simulink model "Ghost_f34"  (Simulink 8.1)
settings: Solver=ode1  StartTime=0.0  StopTime=inf  FixedStep=Ts  MaxStep=1e-3  RelTol=1e-3
PostLoadFcn:
  | NREL_Mode=1; Ghost_init;
InitFcn:
  | NREL_Mode=1; Ghost_init;
values from neighbouring files (symbols this model uses):
  DER_REL = xlsread('DER_relay.xlsx')    [relay_settings_init.m]
  Ts = 100E-6    (= 0.0001)    [BANSHEE_init.m]    (also in Ghost_init.m)
undefined symbols (not defined in the file or in its folder): CBID, Feeder3_lib, Left, SM_UtilityService, SS_Feeder3, Stim, type, utility_service_lib, V
libraries: simulink x72, cables_lib x16, breaker_lib x14, transformer_lib x7, powerlib x7, rtlab x6, Load_lib x6, ssn_lib x4, artemis x2, PHIL_lib x2, rtio_generic_modbus x2, NREL_Diesel_Genset_lib x2
(part 1 of 3)
settings Model: ARTEMISmethode_block_infos=$$__separator__$$Ghost_f34/ARTEMIS Guide$$__separator__$$  Creator=RE25624  LastModifiedBy=hptb1  BufferReuse=off
settings SolverCC: ZeroCrossAlgorithm=Adaptive
settings DataIOCC: ExternalInput=getinputstruct(op_snapshot1)  InitialState=getstatestruct(op_snapshot1)  LimitDataPoints=off  MaxDataPoints=90060  SignalLoggingSaveFormat=Dataset  SaveOutput=off  SignalLogging=off  DSMLogging=off  SaveTime=off  OutputSaveName=result
settings OptimizationCC: BlockReduction=off  OptimizeBlockIOStorage=off  BufferReuse=off  ExpressionFolding=off  LocalBlockOutputs=off
settings DebuggingCC: MaxConsecutiveZCsMsg=warning  IgnoredZcDiagnostic=none  SolverPrmCheckMsg=none  MultiTaskRateTransMsg=warning  ParameterPrecisionLossMsg=none  FcnCallInpInsideContextMsg=EnableAllAsWarning  FrameProcessingCompatibilityMsg=error  ModelReferenceExtraNoncontSigs=warning  StrictBusMsg=Warning
settings ModelReferenceCC: UpdateModelReferenceTargets=IfOutOfDate
settings SFSimCC: SFSimEcho=off
settings GRTTargetCC: CodeReplacementLibrary=C89/C90 (ANSI)

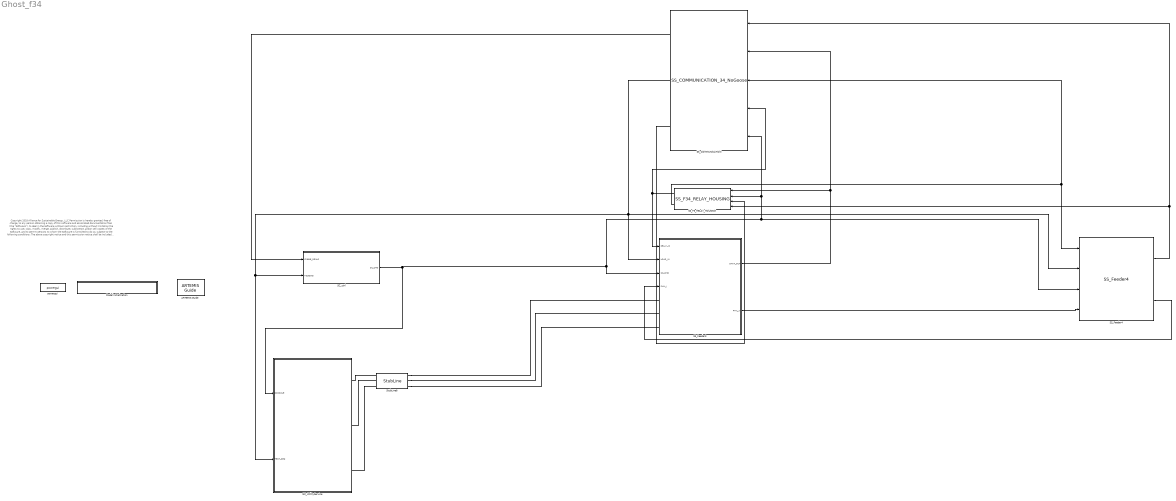
== system Ghost_f34 ==
  note: Copyright 2018 Alliance for Sustainable Energy, LLC
      |
      | Permission is hereby granted, free of charge, to any person obtaining a copy of this software
      | and associated documentation files (the "Software"), to deal in the Software without restriction,
      | including without limitation the rights to use, copy, modify, merge, publish, distribute, sublicense,
      | and/or sell copies of the Software, and to permit persons to whom the Software is furnished to do so,
      | subject to the following conditions:
      |
      | The above copyright notice and this permission notice shall be included in all copies or substantial portions of the Software.
      |
      | THE SOFTWARE IS PROVIDED "AS IS", WITHOUT WARRANTY OF ANY KIND, EXPRESS OR IMPLIED, INCLUDING
      | BUT NOT LIMITED TO THE WARRANTIES OF MERCHANTABILITY, FITNESS FOR A PARTICULAR PURPOSE AND
      | NONINFRINGEMENT. IN NO EVENT SHALL THE AUTHORS, THE COPYRIGHT HOLDERS, THE UNITED STATES,
      | THE UNITED STATES DEPARTMENT OF ENERGY, OR ANY OF THEIR EMPLOYEES BE LIABLE FOR ANY CLAIM,
      | DAMAGES OR OTHER LIABILITY, WHETHER IN AN ACTION OF CONTRACT, TORT OR OTHERWISE, ARISING FROM,
      | OUT OF OR IN CONNECTION WITH THE SOFTWARE OR THE USE OR OTHER DEALINGS IN THE SOFTWARE.
  ARTEMIS Guide : artemis/ARTEMIS/ARTEMIS Guide  Tag=FTSSmethode_opal_4hx0r99  Description=5.0_z1  lock=on  Ts=Ts  opt=art5  dyna=off  nb_perm=4  RT_fullcomp=off  ssn=on  ssn_itvc=off  ssn_ivic=off  ssn_ext=off  ssn_solver=Art5 with Backward Euler nodal interface  ssn_impulse=off  ssn_quasimpulse=off  ssn_impulse_loop=5  paraExtinctionThy=off  Thy_Impulse=on  dtc=Off  dtc_opt=normal  ao=on  simtype=off  ct_mac=off  lin_mov=off  lsp=[0.001 2]  spike_skip=Disabled  dtc_extra=1  dtc_sws=normal  dtc_pied=0.5  SPSRulesBlock=SPSRules  tre=on  ctmm=off  LF=off  dpl_type=ARTEMiS DPL  rlc_type=off  custom_type=off  para=on  ssn_ImpulseLoopBlockedStateUpdate=5  ssn_mov_iter_number=5  ssn_switch_iter_number=5  ssn_nib_type_verify=on
  Model Initialization : Subsystem  AncestorBlock=artemis/Tools /Misc/Model Initialization  mask(Model Functions){InitFcnX=NREL_Mode=1; Ghost_init;, prel=off, posl=on, inif=on, strf=off}
      mask prompts: InitFcnX "Initialisation"; prel "Preload Function"; posl "PostLoad Function"; inif "InitFcn"; strf "StartFcn"
      mask init:
      | currentBlock = gcb;
      | root = bdroot(currentBlock);
      | 
      | if ~strcmp(get_param(root,'BlockDiagramType'),'library')
      |     if prel==1
      |         set_param(root, 'PreLoadFcn', InitFcnX);
      |     else
      |         set_param(root, 'PreLoadFcn', '');
      |     end
      |     if inif==1
      |         set_param(root, 'InitFcn', InitFcnX);
      |     else
      |         set_param(root, 'InitFcn', '');
      |     end
      |     if strf==1
      |         set_param(root, 'StartFcn', InitFcnX);
      |     else
      |         set_param(root, 'StartFcn', '');
      |     end
      |     if posl==1
      |         set_param(root, 'PostLoadFcn', InitFcnX);
      |     else
      |         set_param(root, 'PostLoadFcn', '');
      |     end
      | end
      | 
      | pos = get_param(currentBlock, 'Position');
      | width = pos(3) - pos(1); height = pos(4) - pos(2);
      | txt = [ upper(root) '\n' '- InitFcn. . . . . '  get_param(root, 'InitFcn') ];
      settings: CopyFcn=set_param(gcb,'LinkStatus','inactive')
      mask Display: text(5, height*0.5, txt, 'horizontalAlignment', 'left', 'verticalAlignment', 'middle') ;
  SC_ctrl : Subsystem
  SM_UtilityService : Subsystem  AncestorBlock=utility_service_lib/SM_UtilityService
  SS_COMMUNICATION : communications_lib/SS_COMMUNICATION_34_NoGoose
  SS_F3_RELAY_HOUSING : relay_housing_lib/SS_F34_RELAY_HOUSING
  SS_Feeder3 : Subsystem  AncestorBlock=Feeder3_lib/SS_Feeder3
  SS_Feeder4 : Feeder4_lib/SS_Feeder4
  StubLine8 : artemis/ARTEMIS/StubLine  Phases=3  pu=on  L=1500 * 9.43453e-08 / 2  Lpu=0.08  R=1500 * 2.28409e-5 / 2  Rpu=0.002  S_base=50e6/3  V_base=13.8e3/sqrt(3)  F_base=60  Ts=Ts
  powergui : powerlib/powergui  Priority=2  SimulationMode=Discrete  SolverType=Tustin  SampleTime=Ts  frequency=60  SPID=off  DisableSnubberDevices=off  DisableRonSwitches=off  DisableVfSwitches=off  SwTol=0  Interpol=off  DisplayEquations=off  frequencyindice=0  Pbase=100e6  ErrMax=1e-4  Iterations=50  UnitsV=kV  UnitsW=MW  FunctionMessages=off  echomessages=off  HookPort=off  EnableUseOfTLC=off  x0status=blocks  RestoreLinks=warning  ResistiveCurrentMeasurement=off  Frange=logspace(0,3,50)  Ylog=off  Xlog=off  ShowGrid=off  save=off  variable=ZData  structure=0  ZoomFFT=on  StartTime=0.0  cycles=2  DisplayStyle=off  fundamental=60  FreqAxis=off  MaxFrequency=1000  frequencyindicesteady=1  RmsSteady=1  display=off  Ts=0  methode=off
  wires:
  SS_Feeder3/1(DATA_OUT) -> SS_COMMUNICATION/2, SS_F3_RELAY_HOUSING/1
  SS_F3_RELAY_HOUSING/1 -> SS_COMMUNICATION/4, SS_Feeder3/1(RELAY_IN)
  SS_COMMUNICATION/1 -> SC_ctrl/1(CMBNE_SGNLS)
  SC_ctrl/1(SC_CMD) -> SS_Feeder3/3(SC_CMD), SS_Feeder4/3, SS_COMMUNICATION/5, SS_F3_RELAY_HOUSING/2, SM_UtilityService/1(CONSOLE)
  SS_F3_RELAY_HOUSING/2 -> SS_COMMUNICATION/3, SS_Feeder4/1
  SS_Feeder4/1 -> SS_COMMUNICATION/1, SS_F3_RELAY_HOUSING/4
  SS_Feeder3/2(PHIL_V) -> SS_Feeder4/4
  SS_Feeder4/2 -> SS_Feeder3/4(PHIL_I)
  SS_COMMUNICATION/3 -> SS_F3_RELAY_HOUSING/3
  SS_COMMUNICATION/2 -> SS_Feeder3/2(LOAD_IN), SM_UtilityService/2(TEST_SEQ), SC_ctrl/2(TestData), SS_Feeder4/2
  connections:
  StubLine8/LConn1 -- SM_UtilityService/RConn1
  StubLine8/LConn2 -- SM_UtilityService/RConn2
  StubLine8/LConn3 -- SM_UtilityService/RConn3
  StubLine8/RConn3 -- SS_Feeder3/LConn3
  StubLine8/RConn2 -- SS_Feeder3/LConn2
  StubLine8/RConn1 -- SS_Feeder3/LConn1

== system Ghost_f34/Model Initialization ==

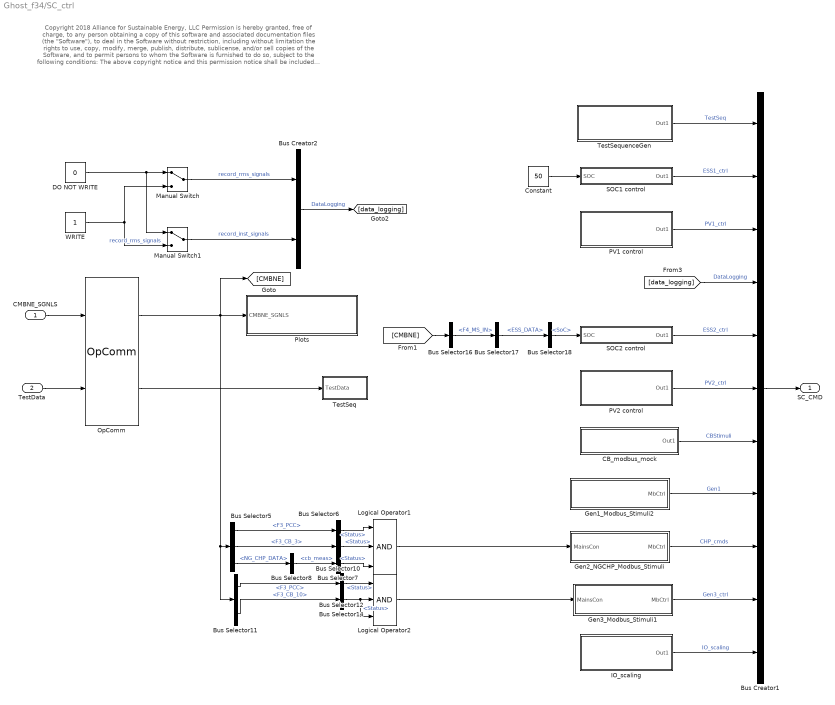
== system Ghost_f34/SC_ctrl ==
  note: Copyright 2018 Alliance for Sustainable Energy, LLC
      |
      | Permission is hereby granted, free of charge, to any person obtaining a copy of this software
      | and associated documentation files (the "Software"), to deal in the Software without restriction,
      | including without limitation the rights to use, copy, modify, merge, publish, distribute, sublicense,
      | and/or sell copies of the Software, and to permit persons to whom the Software is furnished to do so,
      | subject to the following conditions:
      |
      | The above copyright notice and this permission notice shall be included in all copies or substantial portions of the Software.
      |
      | THE SOFTWARE IS PROVIDED "AS IS", WITHOUT WARRANTY OF ANY KIND, EXPRESS OR IMPLIED, INCLUDING
      | BUT NOT LIMITED TO THE WARRANTIES OF MERCHANTABILITY, FITNESS FOR A PARTICULAR PURPOSE AND
      | NONINFRINGEMENT. IN NO EVENT SHALL THE AUTHORS, THE COPYRIGHT HOLDERS, THE UNITED STATES,
      | THE UNITED STATES DEPARTMENT OF ENERGY, OR ANY OF THEIR EMPLOYEES BE LIABLE FOR ANY CLAIM,
      | DAMAGES OR OTHER LIABILITY, WHETHER IN AN ACTION OF CONTRACT, TORT OR OTHERWISE, ARISING FROM,
      | OUT OF OR IN CONNECTION WITH THE SOFTWARE OR THE USE OR OTHER DEALINGS IN THE SOFTWARE.
  CMBNE_SGNLS : Inport
  TestData : Inport  Port=2
  Bus Creator1 : BusCreator  Inputs=11
  Bus Creator2 : BusCreator  Inputs=2
  Bus Selector{6..7,10,12,14} (5 alike) : BusSelector  OutputSignals=Status
  Bus Selector11 : BusSelector  OutputSignals=F3_MS_IN.CB_DATA.F3_PCC,F3_MS_IN.CB_DATA.F3_CB_10
  Bus Selector16 : BusSelector  OutputSignals=F4_MS_IN
  Bus Selector17 : BusSelector  OutputSignals=ESS_DATA
  Bus Selector18 : BusSelector  OutputSignals=Battery.SoC
  Bus Selector5 : BusSelector  OutputSignals=F3_MS_IN.CB_DATA.F3_PCC,F3_MS_IN.CB_DATA.F3_CB_3,F3_MS_IN.NG_CHP_DATA
  Bus Selector8 : BusSelector  OutputSignals=cb.cb_meas
  CB_modbus_mock : Subsystem
  Constant : Constant  Value=50
  DO NOT WRITE : Constant  Value=0
  Gen1_Modbus_Stimuli2 : Subsystem
  Gen2_NGCHP_Modbus_Stimuli : Subsystem
  Gen3_Modbus_Stimuli1 : Subsystem
  IO_scaling : Subsystem
  Logical Operator1 : Logic  Inputs=3  AllPortsSameDT=off  OutDataTypeStr=boolean
  Logical Operator2 : Logic  Inputs=3  AllPortsSameDT=off  OutDataTypeStr=boolean
  Manual Switch : ManualSwitch
  Manual Switch1 : ManualSwitch
  OpComm : rtlab/OpComm  nbport=2  groupe_acq=1  subsys_rate=0  st=0  Synchronization=on  Interpolation=on  Threshold=1.0  Missed_Data=off  Sim_Time=off  Samples=off  dynSigOut=off  from_console=0  warning_done=off  writeOpCommFile=off  Offset=off
  PV1 control : Subsystem
  PV2 control : Subsystem
  Plots : Subsystem
  SOC1 control : Subsystem
  SOC2 control : Subsystem
  TestSeq : Subsystem
  TestSequenceGen : Subsystem
  WRITE : Constant
  SC_CMD : Outport
  wires:
  CMBNE_SGNLS/1 -> OpComm/1
  Bus Creator1/1 -> SC_CMD/1
  Manual Switch/1 -> Bus Creator2/1  "record_rms_signals"
  Manual Switch1/1 -> Bus Creator2/2  "record_inst_signals"
  Bus Creator2/1 -> [data_logging]  "DataLogging"
  TestData/1 -> OpComm/2
  WRITE/1 -> Manual Switch1/2, Manual Switch/2  "record_rms_signals"
  DO NOT WRITE/1 -> Manual Switch1/1, Manual Switch/1
  [data_logging] -> Bus Creator1/4  "DataLogging"
  CB_modbus_mock/1(Out1) -> Bus Creator1/7  "CBStimuli"
  Gen1_Modbus_Stimuli2/1(MbCtrl) -> Bus Creator1/8  "Gen1"
  SOC2 control/1(Out1) -> Bus Creator1/5  "ESS2_ctrl"
  PV2 control/1(Out1) -> Bus Creator1/6  "PV2_ctrl"
  OpComm/1 -> [CMBNE], Bus Selector11/1, Bus Selector5/1, Plots/1(CMBNE_SGNLS)
  Gen2_NGCHP_Modbus_Stimuli/1(MbCtrl) -> Bus Creator1/9  "CHP_cmds"
  Bus Selector5/1 -> Bus Selector6/1  "<F3_PCC>"
  Bus Selector5/3 -> Bus Selector8/1  "<NG_CHP_DATA>"
  Bus Selector6/1 -> Logical Operator1/1  "<Status>"
  Bus Selector7/1 -> Logical Operator1/3  "<Status>"
  Bus Selector8/1 -> Bus Selector7/1  "<cb_meas>"
  Logical Operator1/1 -> Gen2_NGCHP_Modbus_Stimuli/1(MainsCon)
  Bus Selector10/1 -> Logical Operator1/2  "<Status>"
  Bus Selector5/2 -> Bus Selector10/1  "<F3_CB_3>"
  Gen3_Modbus_Stimuli1/1(MbCtrl) -> Bus Creator1/10  "Gen3_ctrl"
  Logical Operator2/1 -> Gen3_Modbus_Stimuli1/1(MainsCon)
  Bus Selector11/1 -> Bus Selector12/1  "<F3_PCC>"
  Bus Selector12/1 -> Logical Operator2/1  "<Status>"
  Bus Selector11/2 -> Bus Selector14/1  "<F3_CB_10>"
  Bus Selector14/1 -> Logical Operator2/3, Logical Operator2/2  "<Status>"
  OpComm/2 -> TestSeq/1(TestData)
  IO_scaling/1(Out1) -> Bus Creator1/11  "IO_scaling"
  TestSequenceGen/1(Out1) -> Bus Creator1/1  "TestSeq"
  SOC1 control/1(Out1) -> Bus Creator1/2  "ESS1_ctrl"
  PV1 control/1(Out1) -> Bus Creator1/3  "PV1_ctrl"
  Constant/1 -> SOC1 control/1(SOC)
  [CMBNE] -> Bus Selector16/1
  Bus Selector16/1 -> Bus Selector17/1  "<F4_MS_IN>"
  Bus Selector17/1 -> Bus Selector18/1  "<ESS_DATA>"
  Bus Selector18/1 -> SOC2 control/1(SOC)  "<SoC>"

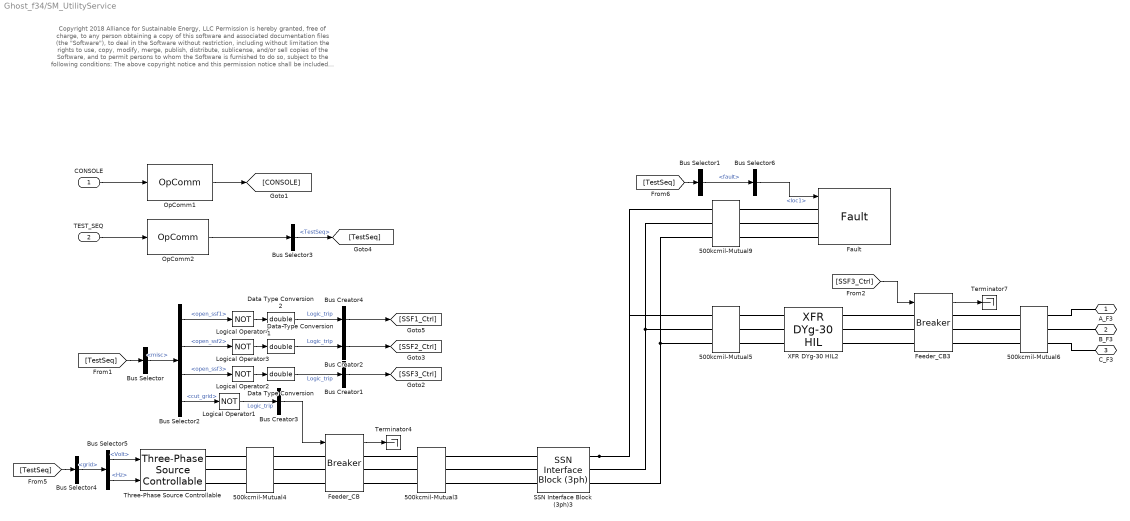
== system Ghost_f34/SM_UtilityService ==
  note: Copyright 2018 Alliance for Sustainable Energy, LLC
      |
      | Permission is hereby granted, free of charge, to any person obtaining a copy of this software
      | and associated documentation files (the "Software"), to deal in the Software without restriction,
      | including without limitation the rights to use, copy, modify, merge, publish, distribute, sublicense,
      | and/or sell copies of the Software, and to permit persons to whom the Software is furnished to do so,
      | subject to the following conditions:
      |
      | The above copyright notice and this permission notice shall be included in all copies or substantial portions of the Software.
      |
      | THE SOFTWARE IS PROVIDED "AS IS", WITHOUT WARRANTY OF ANY KIND, EXPRESS OR IMPLIED, INCLUDING
      | BUT NOT LIMITED TO THE WARRANTIES OF MERCHANTABILITY, FITNESS FOR A PARTICULAR PURPOSE AND
      | NONINFRINGEMENT. IN NO EVENT SHALL THE AUTHORS, THE COPYRIGHT HOLDERS, THE UNITED STATES,
      | THE UNITED STATES DEPARTMENT OF ENERGY, OR ANY OF THEIR EMPLOYEES BE LIABLE FOR ANY CLAIM,
      | DAMAGES OR OTHER LIABILITY, WHETHER IN AN ACTION OF CONTRACT, TORT OR OTHERWISE, ARISING FROM,
      | OUT OF OR IN CONNECTION WITH THE SOFTWARE OR THE USE OR OTHER DEALINGS IN THE SOFTWARE.
  CONSOLE : Inport
  TEST_SEQ : Inport  Port=2
  500kcmil-Mutual3 : cables_lib/500kcmil-Mutual  length=50  par_sets=1  ratio=3
  500kcmil-Mutual4 : cables_lib/500kcmil-Mutual  length=50  par_sets=1  ratio=3
  500kcmil-Mutual5 : cables_lib/500kcmil-Mutual  length=200  par_sets=1  ratio=3
  500kcmil-Mutual6 : cables_lib/500kcmil-Mutual  length=50  par_sets=1  ratio=3
  500kcmil-Mutual9 : cables_lib/500kcmil-Mutual  length=200  par_sets=1  ratio=3
  Bus Creator{1..4} (4 alike) : BusCreator  Inputs=1
  Bus Selector : BusSelector  OutputSignals=misc
  Bus Selector1 : BusSelector  OutputSignals=fault
  Bus Selector2 : BusSelector  OutputSignals=open_ssf1,open_ssf2,open_ssf3,cut_grid
  Bus Selector3 : BusSelector  OutputSignals=TestSeq
  Bus Selector4 : BusSelector  OutputSignals=grid
  Bus Selector5 : BusSelector  OutputSignals=Volt,Hz
  Bus Selector6 : BusSelector  OutputSignals=loc1
  Data Type Conversion : DataTypeConversion  OutDataTypeStr=double
  Data Type Conversion1 : DataTypeConversion  OutDataTypeStr=double
  Data Type Conversion2 : DataTypeConversion  OutDataTypeStr=double
  Fault : fault_lib/Fault  FaultResistance=0.1  GroundResistance=1.73  SnubberResistance=1E6
  Feeder_CB : breaker_lib/Breaker  Ts=Ts  mech_delay=cb_mech_delay
  Feeder_CB3 : breaker_lib/Breaker  Ts=Ts  mech_delay=cb_mech_delay
  Logical Operator{1..4} (4 alike) : Logic  Operator=NOT  AllPortsSameDT=off  OutDataTypeStr=boolean
  OpComm1 : rtlab/OpComm  nbport=1  groupe_acq=1  subsys_rate=0  st=0  Synchronization=on  Interpolation=on  Threshold=1.0  Missed_Data=off  Sim_Time=off  Samples=off  dynSigOut=off  from_console=1  warning_done=off  writeOpCommFile=off  Offset=off
  OpComm2 : rtlab/OpComm  nbport=1  groupe_acq=1  subsys_rate=0  st=0  Synchronization=on  Interpolation=on  Threshold=1.0  Missed_Data=off  Sim_Time=off  Samples=off  dynSigOut=off  from_console=0  warning_done=off  writeOpCommFile=off  Offset=off
  SSN Interface Block (3ph)3 : ssn_lib/SSN Interface Block (3ph)  nb_phase=3  nb_port=2  p1_type=V-type(Left)  p2_type=V-type (Right)  p3_type=V-type(Left)  p4_type=V-type(Left)  p5_type=V-type(Left)  p6_type=V-type(Left)  p7_type=V-type(Left)  p8_type=V-type(Left)  p9_type=V-type(Left)  p10_type=V-type(Left)  p11_type=V-type(Left)  p12_type=V-type(Left)  p13_type=V-type(Left)  p14_type=V-type(Left)  p15_type=V-type(Left)  p16_type=V-type(Left)  I_port_shunt_resistance=1e9
  Terminator4 : Terminator
  Terminator7 : Terminator
  Three-Phase Source Controllable : controllable_grid_lib/Three-Phase Source Controllable  Ts=Ts  Rg=0.8  Lg=16.58e-3  mask{Ts=Ts}
  XFR DYg-30 HIL2 : transformer_lib/XFR DYg-30 HIL  Rating=50000  Vp=115000  Vs=13800  Z=6  XR=30
  A_F3 : PMIOPort  Port=1  Side=Right
  B_F3 : PMIOPort  Port=2  Side=Right
  C_F3 : PMIOPort  Port=3  Side=Right
  wires:
  CONSOLE/1 -> OpComm1/1
  OpComm1/1 -> [CONSOLE]
  Feeder_CB/1 -> Terminator4/1
  Feeder_CB3/1 -> Terminator7/1
  TEST_SEQ/1 -> OpComm2/1
  [TestSeq] -> Bus Selector/1
  Logical Operator1/1 -> Bus Creator3/1  "Logic_trip"
  Bus Creator3/1 -> Feeder_CB/1
  Bus Selector/1 -> Bus Selector2/1  "<misc>"
  Bus Selector2/4 -> Logical Operator1/1  "<cut_grid>"
  Bus Selector2/3 -> Logical Operator2/1  "<open_ssf3>"
  Logical Operator2/1 -> Data Type Conversion/1
  Bus Creator1/1 -> [SSF3_Ctrl]
  Data Type Conversion/1 -> Bus Creator1/1  "Logic_trip"
  Bus Selector3/1 -> [TestSeq]  "<TestSeq>"
  OpComm2/1 -> Bus Selector3/1
  Bus Selector2/2 -> Logical Operator3/1  "<open_ssf2>"
  Logical Operator3/1 -> Data Type Conversion1/1
  Bus Creator2/1 -> [SSF2_Ctrl]
  Data Type Conversion1/1 -> Bus Creator2/1  "Logic_trip"
  Bus Selector2/1 -> Logical Operator4/1  "<open_ssf1>"
  Logical Operator4/1 -> Data Type Conversion2/1
  Bus Creator4/1 -> [SSF1_Ctrl]
  Data Type Conversion2/1 -> Bus Creator4/1  "Logic_trip"
  [SSF3_Ctrl] -> Feeder_CB3/1
  [TestSeq] -> Bus Selector4/1
  Bus Selector4/1 -> Bus Selector5/1  "<grid>"
  Bus Selector5/2 -> Three-Phase Source Controllable/2  "<Hz>"
  Bus Selector5/1 -> Three-Phase Source Controllable/1  "<Volt>"
  [TestSeq] -> Bus Selector1/1
  Bus Selector1/1 -> Bus Selector6/1  "<fault>"
  Bus Selector6/1 -> Fault/1  "<loc1>"
  connections:
  500kcmil-Mutual3/LConn3 -- Feeder_CB/RConn3
  500kcmil-Mutual3/LConn1 -- Feeder_CB/RConn1
  500kcmil-Mutual3/LConn2 -- Feeder_CB/RConn2
  SSN Interface Block (3ph)3/LConn2 -- 500kcmil-Mutual3/RConn2
  SSN Interface Block (3ph)3/LConn1 -- 500kcmil-Mutual3/RConn1
  SSN Interface Block (3ph)3/LConn3 -- 500kcmil-Mutual3/RConn3
  500kcmil-Mutual4/RConn3 -- Feeder_CB/LConn3
  500kcmil-Mutual4/RConn2 -- Feeder_CB/LConn2
  500kcmil-Mutual4/RConn1 -- Feeder_CB/LConn1
  Three-Phase Source Controllable/RConn3 -- 500kcmil-Mutual4/LConn3
  Three-Phase Source Controllable/RConn1 -- 500kcmil-Mutual4/LConn1
  Three-Phase Source Controllable/RConn2 -- 500kcmil-Mutual4/LConn2
  500kcmil-Mutual5/RConn2 -- XFR DYg-30 HIL2/LConn2
  500kcmil-Mutual5/RConn1 -- XFR DYg-30 HIL2/LConn1
  500kcmil-Mutual5/RConn3 -- XFR DYg-30 HIL2/LConn3
  SSN Interface Block (3ph)3/RConn1 -- 500kcmil-Mutual5/LConn1 -- 500kcmil-Mutual9/LConn1
  500kcmil-Mutual5/LConn2 -- SSN Interface Block (3ph)3/RConn2 -- 500kcmil-Mutual9/LConn2
  500kcmil-Mutual5/LConn3 -- SSN Interface Block (3ph)3/RConn3 -- 500kcmil-Mutual9/LConn3
  XFR DYg-30 HIL2/RConn1 -- Feeder_CB3/LConn1
  XFR DYg-30 HIL2/RConn2 -- Feeder_CB3/LConn2
  XFR DYg-30 HIL2/RConn3 -- Feeder_CB3/LConn3
  500kcmil-Mutual6/LConn2 -- Feeder_CB3/RConn2
  500kcmil-Mutual6/LConn3 -- Feeder_CB3/RConn3
  500kcmil-Mutual6/LConn1 -- Feeder_CB3/RConn1
  B_F3/RConn1 -- 500kcmil-Mutual6/RConn2
  A_F3/RConn1 -- 500kcmil-Mutual6/RConn1
  C_F3/RConn1 -- 500kcmil-Mutual6/RConn3
  500kcmil-Mutual9/RConn2 -- Fault/LConn2
  500kcmil-Mutual9/RConn3 -- Fault/LConn3
  500kcmil-Mutual9/RConn1 -- Fault/LConn1

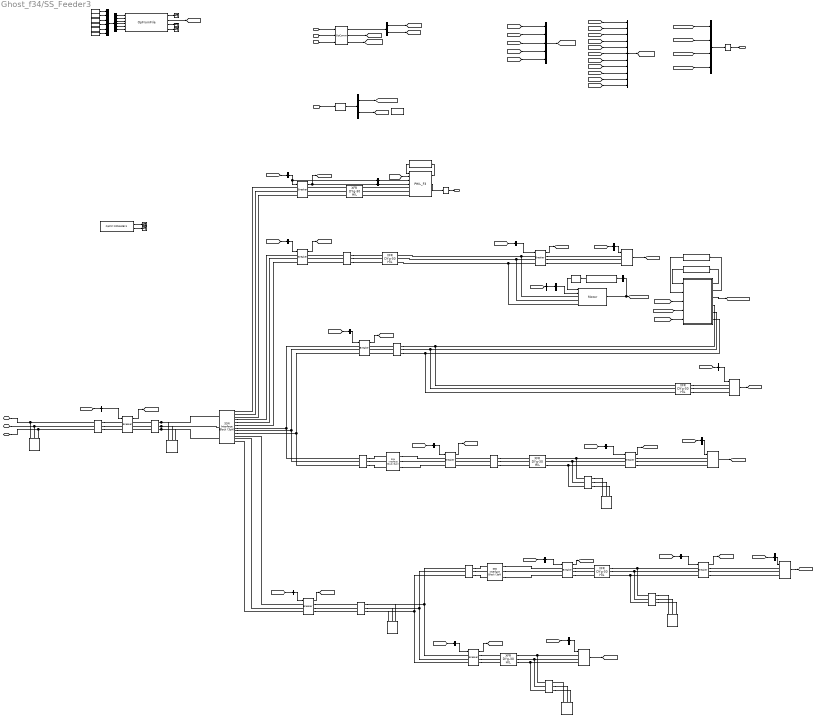
== system Ghost_f34/SS_Feeder3 ==
  note: Signal for this Cb will come from a SEL relay
  note: connect to F2
  note: connect to F2
  note: PHIL interface
  note: Copyright 2018 Alliance for Sustainable Energy, LLC
      |
      | Permission is hereby granted, free of charge, to any person obtaining a copy of this software
      | and associated documentation files (the "Software"), to deal in the Software without restriction,
      | including without limitation the rights to use, copy, modify, merge, publish, distribute, sublicense,
      | and/or sell copies of the Software, and to permit persons to whom the Software is furnished to do so,
      | subject to the following conditions:
      |
      | The above copyright notice and this permission notice shall be included in all copies or substantial portions of the Software.
      |
      | THE SOFTWARE IS PROVIDED "AS IS", WITHOUT WARRANTY OF ANY KIND, EXPRESS OR IMPLIED, INCLUDING
      | BUT NOT LIMITED TO THE WARRANTIES OF MERCHANTABILITY, FITNESS FOR A PARTICULAR PURPOSE AND
      | NONINFRINGEMENT. IN NO EVENT SHALL THE AUTHORS, THE COPYRIGHT HOLDERS, THE UNITED STATES,
      | THE UNITED STATES DEPARTMENT OF ENERGY, OR ANY OF THEIR EMPLOYEES BE LIABLE FOR ANY CLAIM,
      | DAMAGES OR OTHER LIABILITY, WHETHER IN AN ACTION OF CONTRACT, TORT OR OTHERWISE, ARISING FROM,
      | OUT OF OR IN CONNECTION WITH THE SOFTWARE OR THE USE OR OTHER DEALINGS IN THE SOFTWARE.
  RELAY_IN : Inport
  LOAD_IN : Inport  Port=2
  SC_CMD : Inport  Port=3
  PHIL_I : Inport  Port=4
  1000 kVA : transformer_lib/XFR DYg-30 HIL  Rating=1000  Vp=13800  Vs=480  Z=5.56  XR=5.49
  1000 kVA1 : transformer_lib/XFR DYg-30 HIL  Rating=1000  Vp=13800  Vs=480  Z=5.56  XR=5.49
  200 HP chiller compressor : Load_lib/200 HP chiller compressor
  2000 kVA : transformer_lib/XFR DYg-30 HIL  Rating=2000  Vp=13800  Vs=480  Z=5.75  XR=5.7
  2000 kVA1 : transformer_lib/XFR DYg-30 HIL  Rating=2000  Vp=13800  Vs=480  Z=5.75  XR=5.7
  2500 kVA : transformer_lib/XFR DYg-30 HIL  Rating=2500  Vp=13800  Vs=480  Z=5.75  XR=6.6
  2500 kVA1 : transformer_lib/XFR DYg-30 HIL  Rating=5000  Vp=13800  Vs=4160  Z=5.75  XR=6.6
  448 kvar inductor at 13.8kV  to cancel kvar produced by the stublines1 : powerlib/Elements/Three-Phase Parallel RLC Load  LConnTagsString=A|B|C  Configuration=Y (grounded)  NominalVoltage=13800  NominalFrequency=60  ActivePower=10e3  InductivePower=448e3  CapacitivePower=0  Measurements=None  LoadType=constant Z
  500kcmil-Mutual1 : cables_lib/500kcmil-Mutual  length=10  par_sets=1  ratio=3
  500kcmil-Mutual2 : cables_lib/500kcmil-Mutual  length=10  par_sets=1  ratio=3
  500kcmil-Mutual3 : cables_lib/500kcmil-Mutual  length=100  par_sets=1  ratio=3
  500kcmil-Mutual4 : cables_lib/500kcmil-Mutual  length=10  par_sets=1  ratio=3
  500kcmil-Mutual5 : cables_lib/500kcmil-Mutual  length=1000  par_sets=1  ratio=3
  6 kvar inductor at 480V  to cancel kvar produced by the stublines1 : powerlib/Elements/Three-Phase Parallel RLC Load  LConnTagsString=A|B|C  Configuration=Y (grounded)  NominalVoltage=480  NominalFrequency=60  ActivePower=1e3  InductivePower=6e3  CapacitivePower=0  Measurements=None  LoadType=constant Z
  6 kvar inductor at 480V  to cancel kvar produced by the stublines2 : powerlib/Elements/Three-Phase Parallel RLC Load  LConnTagsString=A|B|C  Configuration=Y (grounded)  NominalVoltage=480  NominalFrequency=60  ActivePower=1e3  InductivePower=6e3  CapacitivePower=0  Measurements=None  LoadType=constant Z
  6 kvar inductor at 480V  to cancel kvar produced by the stublines3 : powerlib/Elements/Three-Phase Parallel RLC Load  LConnTagsString=A|B|C  Configuration=Y (grounded)  NominalVoltage=480  NominalFrequency=60  ActivePower=0  InductivePower=6e3  CapacitivePower=0  Measurements=None  LoadType=constant Z
  AIN_AOUT_OP5142EX1 : PHIL_lib/AIN_AOUT_OP5142EX1
  Bus Creator2 : BusCreator
  Bus Creator3 : BusCreator  Inputs=5
  Bus Creator5 : BusCreator  Inputs=11
  Bus Selector : BusSelector  OutputSignals=motor
  Bus Selector1 : BusSelector  OutputSignals=F3_CB_4
  Bus Selector10 : BusSelector  OutputSignals=F3_CB_5
  Bus Selector11 : BusSelector  OutputSignals=P6
  Bus Selector12 : BusSelector  OutputSignals=F3_CB_9
  Bus Selector13 : BusSelector  OutputSignals=F3_CB_3
  Bus Selector14 : BusSelector  OutputSignals=F3_CB_8
  Bus Selector15 : BusSelector  OutputSignals=CHP_cmds,IO_scaling
  Bus Selector16 : BusSelector  OutputSignals=Status
  Bus Selector17 : BusSelector  OutputSignals=RPM
  Bus Selector18 : BusSelector  OutputSignals=LoadProfile,TestSeq
  Bus Selector19 : BusSelector  OutputSignals=Logic_trip
  Bus Selector2 : BusSelector  OutputSignals=C6
  Bus Selector20 : BusSelector  OutputSignals=ena2
  Bus Selector21 : BusSelector  OutputSignals=F3_PCC
  Bus Selector22 : BusSelector  OutputSignals=F3_CB_10
  Bus Selector3 : BusSelector  OutputSignals=P4
  Bus Selector4 : BusSelector  OutputSignals=I6
  Bus Selector5 : BusSelector  OutputSignals=C5
  Bus Selector6 : BusSelector  OutputSignals=F3_CB_2
  Bus Selector7 : BusSelector  OutputSignals=F3_CB_7
  Bus Selector8 : BusSelector  OutputSignals=F3_CB_6
  Bus Selector9 : BusSelector  OutputSignals=F3_CB_1
  C1 : cables_lib/500kcmil-Mutual  length=10  par_sets=1  ratio=3
  C2 : cables_lib/500kcmil-Mutual  length=10  par_sets=1  ratio=3
  C301 : cables_lib/500kcmil-Mutual  length=2500  par_sets=1  ratio=3
  C302 : cables_lib/4//0AWG-Mutual  length=2000  par_sets=1  ratio=3
  C303 : cables_lib/500kcmil-Mutual  length=2000  par_sets=1  ratio=3
  C304 : cables_lib/4//0AWG-Mutual  length=1500  par_sets=2  ratio=3
  CHP_Modbus : rtio_generic_modbus/Modbus device  conf_name=CHP_modbus.opal  conf_name_mask=CHP_modbus.xls  sample_time=Ts
  Critical_5 : Load_lib/Dynamic_Load  V=480  kVA=1000  PF=0.9  Ts=Ts
  Critical_6 : Load_lib/Dynamic_Load  V=480  kVA=800  PF=0.9  Ts=Ts
  Demux2 : Demux  Outputs=6
  F3_CB_{1..6,8..11} (10 alike) : breaker_lib/Breaker  Ts=Ts  mech_delay=cb_mech_delay
  F3_PCC : breaker_lib/Breaker  Ts=Ts  mech_delay=cb_mech_delay
  First-Order Filter : powerlib_meascontrol/Filters/First-Order Filter  FilterType=Lowpass  Tc=10e-3  Ts=Ts  Initialize=on  Vac_Init=[0, 0, 60]  Vdc_Init=0  PlotResponse=off  FreqRange="[0,  200,  1]"
  GEN2_Modbus : rtio_generic_modbus/Modbus device  conf_name=GEN2_modbus.opal  conf_name_mask=GEN2_modbus.xls  sample_time=Ts
  Goto Tag Visibility : GotoTagVisibility  GotoTag=phil_ctrl
  "Interpolation " : Constant
  Interruptible_6 : Load_lib/Dynamic_Load  V=480  kVA=600  PF=0.9  Ts=Ts
  Losses1 : powerlib/Elements/Three-Phase Parallel RLC Load  LConnTagsString=A|B|C  Configuration=Y (grounded)  NominalVoltage=13800  NominalFrequency=60  ActivePower=1e3  InductivePower=0  CapacitivePower=0  Measurements=None  LoadType=constant Z
  Losses4 : powerlib/Elements/Three-Phase Parallel RLC Load  LConnTagsString=A|B|C  Configuration=Y (grounded)  NominalVoltage=13800  NominalFrequency=60  ActivePower=1e3  InductivePower=0  CapacitivePower=0  Measurements=None  LoadType=constant Z
  Memory : Memory
  Memory1 : Memory
  Motor : Motor_InductionMachine_lib/Motor
  Mux : Mux  Inputs=6
  NGCHP_Generator : Subsystem
  OpComm1 : rtlab/OpComm  nbport=3  groupe_acq=1  subsys_rate=0  st=0  Synchronization=on  Interpolation=on  Threshold=1.0  Missed_Data=off  Sim_Time=off  Samples=off  dynSigOut=off  from_console=0  warning_done=off  writeOpCommFile=off  Offset=off
  OpComm2 : rtlab/OpComm  nbport=1  groupe_acq=1  subsys_rate=0  st=0  Synchronization=on  Interpolation=on  Threshold=1.0  Missed_Data=off  Sim_Time=off  Samples=off  dynSigOut=off  from_console=1  warning_done=off  writeOpCommFile=off  Offset=off
  OpCtrl OP5142EX1 : rtio_opalrt_op5142ex1/OpCtrl OP5142EX1  CtrlName='OP5142EX1 Ctrl'  boardid=0  BitstreamFilename=OP5142_1-EX-0000-2_1-96IO-04-01.bin  numconfig=-1  mode=Master  externalClock=off  decimRtsi=0  calibIO=off  SampleTime=0  loadinport=-1
  OpFromFile : rtlab/DataLogging/OpFromFile  filename_mode=Static (same filename all the time)  reload_mode=Next time model is paused (Real-Time)  init_file_id=0  filename=HeatLoad.mat  rtpath='./'  nrtpath='.\'  sample_time=Ts
  PHIL_F3 : PHIL_lib/PHIL_F3
  Priority_4 : Load_lib/Dynamic_Load  V=480  kVA=600  PF=0.9  Ts=Ts
  Priority_6 : Load_lib/Dynamic_Load  V=480  kVA=1000  PF=0.9  Ts=Ts
  "Repetative " : Constant
  SSN Interface Block (3ph)1 : ssn_lib/SSN Interface Block (3ph)  nb_phase=3  nb_port=2  p1_type=V-type(Left)  p2_type=V-type (Right)  p3_type=V-type(Left)  p4_type=V-type(Left)  p5_type=V-type(Left)  p6_type=V-type(Left)  p7_type=V-type(Left)  p8_type=V-type(Left)  p9_type=V-type(Left)  p10_type=V-type(Left)  p11_type=V-type(Left)  p12_type=V-type(Left)  p13_type=V-type(Left)  p14_type=V-type(Left)  p15_type=V-type(Left)  p16_type=V-type(Left)  I_port_shunt_resistance=1e9
  SSN Interface Block (3ph)2 : ssn_lib/SSN Interface Block (3ph)  nb_phase=3  nb_port=2  p1_type=V-type(Left)  p2_type=V-type (Right)  p3_type=V-type(Left)  p4_type=V-type(Left)  p5_type=V-type(Left)  p6_type=V-type(Left)  p7_type=V-type(Left)  p8_type=V-type(Left)  p9_type=V-type(Left)  p10_type=V-type(Left)  p11_type=V-type(Left)  p12_type=V-type(Left)  p13_type=V-type(Left)  p14_type=V-type(Left)  p15_type=V-type(Left)  p16_type=V-type(Left)  I_port_shunt_resistance=1e9
  SSN Interface Block (3ph)5 : ssn_lib/SSN Interface Block (3ph)  nb_phase=3  nb_port=5  p1_type=V-type(Left)  p2_type=V-type (Right)  p3_type=V-type (Right)  p4_type=V-type (Right)  p5_type=V-type (Right)  p6_type=V-type(Left)  p7_type=V-type(Left)  p8_type=V-type(Left)  p9_type=V-type(Left)  p10_type=V-type(Left)  p11_type=V-type(Left)  p12_type=V-type(Left)  p13_type=V-type(Left)  p14_type=V-type(Left)  p15_type=V-type(Left)  p16_type=V-type(Left)  I_port_shunt_resistance=1e9
  "Start_Index " : Constant
  "State " : Constant
  "Stop_Index " : Constant  Value=1800-1
  Terminator{,1..4} (5 alike) : Terminator
  "Time_Scale_Factor " : Constant
  PCC_A : PMIOPort  Port=1  Side=Left
  PCC_B : PMIOPort  Port=2  Side=Left
  PCC_C : PMIOPort  Port=3  Side=Left
  DATA_OUT : Outport
  PHIL_V : Outport  Port=2
  tag scope: phil_ctrl=scoped
  wires:
  Bus Selector1/1 -> F3_CB_4/1  "<F3_CB_4>"
  LOAD_IN/1 -> OpComm1/1
  OpComm1/1 -> Bus Selector18/1
  [LOAD_IN] -> Bus Selector2/1
  [LOAD_IN] -> Bus Selector3/1
  [LOAD_IN] -> Bus Selector4/1
  [LOAD_IN] -> Bus Selector5/1
  Bus Selector2/1 -> Critical_6/1  "<C6>"
  Bus Selector3/1 -> Priority_4/1  "<P4>"
  Bus Selector4/1 -> Interruptible_6/1  "<I6>"
  Bus Selector5/1 -> Critical_5/1  "<C5>"
  Critical_6/1 -> [LOAD_C6]
  Priority_4/1 -> [LOAD_P4]
  Interruptible_6/1 -> [LOAD_I6]
  Critical_5/1 -> [LOAD_C5]
  [LOAD_C6] -> Bus Creator3/2  "F3_C6"
  [LOAD_C5] -> Bus Creator3/1  "F3_C5"
  [LOAD_I6] -> Bus Creator3/3  "F3_I6"
  [LOAD_P4] -> Bus Creator3/4  "F3_P4"
  Bus Creator3/1 -> [LOAD_DATA]  "LOAD"
  F3_CB_4/1 -> [F3_CB_4]
  F3_CB_3/1 -> [F3_CB_3]
  F3_CB_2/1 -> [F3_CB_2]
  F3_CB_6/1 -> [F3_CB_6]
  F3_CB_1/1 -> [F3_CB_1]
  F3_CB_5/1 -> [F3_CB_5]
  [F3_CB_1] -> Bus Creator5/1  "F3_CB_1"
  [F3_CB_5] -> Bus Creator5/5  "F3_CB_5"
  [F3_CB_7] -> Bus Creator5/7  "F3_CB_7"
  [F3_CB_6] -> Bus Creator5/6  "F3_CB_6"
  [F3_CB_3] -> Bus Creator5/3  "F3_CB_3"
  [F3_CB_2] -> Bus Creator5/2  "F3_CB_2"
  [F3_CB_4] -> Bus Creator5/4  "F3_CB_4"
  Bus Creator5/1 -> [CB_DATA]
  [RELAY_IN] -> Bus Selector1/1
  RELAY_IN/1 -> OpComm1/2
  OpComm1/2 -> [RELAY_IN]
  Bus Selector6/1 -> F3_CB_2/1  "<F3_CB_2>"
  [RELAY_IN] -> Bus Selector6/1
  Bus Selector7/1 -> F3_CB_11/1  "<F3_CB_7>"
  [RELAY_IN] -> Bus Selector7/1
  Bus Selector8/1 -> F3_CB_6/1  "<F3_CB_6>"
  [RELAY_IN] -> Bus Selector8/1
  Bus Selector9/1 -> F3_CB_1/1  "<F3_CB_1>"
  [RELAY_IN] -> Bus Selector9/1
  Bus Selector10/1 -> F3_CB_5/1  "<F3_CB_5>"
  [RELAY_IN] -> Bus Selector10/1
  Bus Selector13/1 -> F3_CB_3/1  "<F3_CB_3>"
  [RELAY_IN] -> Bus Selector13/1
  F3_CB_11/1 -> [F3_CB_7]
  F3_PCC/1 -> [F3_PCC]
  [F3_PCC] -> Bus Creator5/11  "F3_PCC"
  [LOAD_IN] -> Bus Selector11/1
  Bus Selector11/1 -> Priority_6/1  "<P6>"
  Priority_6/1 -> [LOAD_P6]
  [LOAD_P6] -> Bus Creator3/5  "F3_P6"
  F3_CB_9/1 -> [F3_CB_9]
  Bus Selector12/1 -> F3_CB_9/1  "<F3_CB_9>"
  [RELAY_IN] -> Bus Selector12/1
  F3_CB_8/1 -> [F3_CB_8]
  Bus Selector14/1 -> F3_CB_8/1  "<F3_CB_8>"
  [RELAY_IN] -> Bus Selector14/1
  [F3_CB_8] -> Bus Creator5/8  "F3_CB_8"
  [F3_CB_9] -> Bus Creator5/9  "F3_CB_9"
  SC_CMD/1 -> OpComm2/1
  Memory/1 -> DATA_OUT/1
  "Start_Index "/1 -> Mux/3
  "Time_Scale_Factor "/1 -> Mux/5
  "State "/1 -> Mux/1
  Demux2/1 -> OpFromFile/1
  Demux2/4 -> OpFromFile/4
  OpFromFile/2 -> [heat_load]  "Heat Load MBtu/hr"
  Demux2/5 -> OpFromFile/5
  "Repetative "/1 -> Mux/2
  Demux2/3 -> OpFromFile/3
  Demux2/6 -> OpFromFile/6
  Demux2/2 -> OpFromFile/2
  Mux/1 -> Demux2/1
  "Interpolation "/1 -> Mux/6
  "Stop_Index "/1 -> Mux/4
  OpComm2/1 -> Bus Selector15/1
  Bus Creator2/1 -> Memory/1
  [CB_DATA] -> Bus Creator2/1  "CB_DATA"
  [LOAD_DATA] -> Bus Creator2/2  "LOAD_DATA"
  [NG_CHP_DATA] -> Bus Creator2/3  "NG_CHP_DATA"
  Bus Selector17/1 -> 200 HP chiller compressor/1  "<RPM>"
  200 HP chiller compressor/1 -> First-Order Filter/1
  [TestSeq] -> Bus Selector/1
  Bus Selector/1 -> Bus Selector20/1  "<motor>"
  Bus Selector21/1 -> F3_PCC/1  "<F3_PCC>"
  [RELAY_IN] -> Bus Selector21/1
  [NGCHP_Gen] -> NGCHP_Generator/3(console)
  GEN2_Modbus/1 -> NGCHP_Generator/1(ModbusIn)
  NGCHP_Generator/1(ModbusOut) -> GEN2_Modbus/1  "Gen_meas"
  NGCHP_Generator/3(Gen_meas) -> [NG_CHP_DATA]
  [heat_load] -> NGCHP_Generator/4(Heat Load MBtu/hrs)
  NGCHP_Generator/2(ModbusOutCHP) -> CHP_Modbus/1
  CHP_Modbus/1 -> NGCHP_Generator/2(ModbusIn1)
  Bus Selector15/1 -> [NGCHP_Gen]  "<CHP_cmds>"
  [RELAY_IN] -> Bus Selector22/1
  [F3_CB_10] -> Bus Creator5/10  "F3_CB_10"
  OpComm1/3 -> [PHIL_I]
  PHIL_I/1 -> OpComm1/3
  Bus Selector18/1 -> [LOAD_IN]  "<LoadProfile>"
  Bus Selector18/2 -> [TestSeq]  "<TestSeq>"
  F3_CB_10/1 -> Bus Selector16/1, [F3_CB_10]
  Bus Selector22/1 -> Bus Selector19/1, F3_CB_10/1  "<F3_CB_10>"
  Memory1/1 -> PHIL_V/1
  Bus Selector16/1 -> PHIL_F3/4  "<Status>"
  PHIL_F3/2 -> Memory1/1
  Bus Selector19/1 -> PHIL_F3/3  "<Logic_trip>"
  [PHIL_I] -> PHIL_F3/2
  Bus Selector20/1 -> Motor/2  "<ena2>"
  Bus Selector15/2 -> [phil_ctrl]  "<IO_scaling>"
  OpFromFile/4 -> Terminator2/1
  OpFromFile/1 -> Terminator3/1
  OpFromFile/3 -> Terminator4/1
  Motor/1 -> Bus Selector17/1, [MOTOR_DATA]
  [MOTOR_DATA] -> Bus Creator2/4  "MOTOR_DATA"
  [TestSeq] -> NGCHP_Generator/5(testseq)
  First-Order Filter/1 -> Motor/1
  OpCtrl OP5142EX1/1 -> Terminator/1
  OpCtrl OP5142EX1/2 -> Terminator1/1
  PHIL_F3/1 -> AIN_AOUT_OP5142EX1/1
  AIN_AOUT_OP5142EX1/1 -> PHIL_F3/1
  connections:
  C1/LConn1 -- F3_CB_5/LConn1 -- C301/RConn1 -- Losses1/LConn3
  F3_CB_6/RConn3 -- 2000 kVA1/LConn3
  C1/LConn3 -- F3_CB_5/LConn3 -- C301/RConn3 -- Losses1/LConn1
  C304/LConn1 -- F3_CB_2/RConn1
  C302/RConn3 -- NGCHP_Generator/RConn3 -- 1000 kVA1/LConn3
  C302/LConn2 -- F3_CB_3/RConn2
  C302/RConn1 -- 1000 kVA1/LConn1 -- NGCHP_Generator/RConn1
  F3_CB_6/RConn2 -- 2000 kVA1/LConn2
  C302/RConn2 -- 1000 kVA1/LConn2 -- NGCHP_Generator/RConn2
  F3_CB_5/RConn2 -- 2000 kVA/LConn2
  C302/LConn3 -- F3_CB_3/RConn3
  C1/LConn2 -- F3_CB_5/LConn2 -- C301/RConn2 -- Losses1/LConn2
  C304/LConn2 -- F3_CB_2/RConn2
  F3_CB_6/RConn1 -- 2000 kVA1/LConn1
  C302/LConn1 -- F3_CB_3/RConn1
  F3_CB_5/RConn1 -- 2000 kVA/LConn1
  F3_CB_5/RConn3 -- 2000 kVA/LConn3
  C304/LConn3 -- F3_CB_2/RConn3
  F3_CB_11/RConn1 -- Priority_4/LConn1
  F3_CB_11/RConn3 -- Priority_4/LConn3
  F3_CB_11/RConn2 -- Priority_4/LConn2
  2000 kVA1/RConn1 -- 500kcmil-Mutual2/LConn1 -- F3_CB_8/LConn1
  500kcmil-Mutual2/LConn3 -- 2000 kVA1/RConn3 -- F3_CB_8/LConn3
  2000 kVA1/RConn2 -- 500kcmil-Mutual2/LConn2 -- F3_CB_8/LConn2
  2000 kVA/RConn1 -- 500kcmil-Mutual1/LConn1 -- Critical_5/LConn1
  2000 kVA/RConn3 -- 500kcmil-Mutual1/LConn3 -- Critical_5/LConn3
  2000 kVA/RConn2 -- 500kcmil-Mutual1/LConn2 -- Critical_5/LConn2
  Motor/LConn1 -- 2500 kVA/RConn1 -- F3_CB_9/LConn1
  Motor/LConn3 -- F3_CB_9/LConn3 -- 2500 kVA/RConn3
  Motor/LConn2 -- 2500 kVA/RConn2 -- F3_CB_9/LConn2
  C304/RConn2 -- 1000 kVA/LConn2
  C304/RConn3 -- 1000 kVA/LConn3
  C304/RConn1 -- 1000 kVA/LConn1
  500kcmil-Mutual4/LConn2 -- 1000 kVA/RConn2 -- F3_CB_11/LConn2
  500kcmil-Mutual4/LConn1 -- F3_CB_11/LConn1 -- 1000 kVA/RConn1
  F3_CB_9/RConn1 -- Priority_6/LConn1
  F3_CB_9/RConn2 -- Priority_6/LConn2
  F3_CB_9/RConn3 -- Priority_6/LConn3
  F3_CB_8/RConn1 -- Interruptible_6/LConn1
  F3_CB_8/RConn2 -- Interruptible_6/LConn2
  F3_CB_8/RConn3 -- Interruptible_6/LConn3
  SSN Interface Block (3ph)5/RConn4 -- F3_CB_4/LConn1
  SSN Interface Block (3ph)5/RConn6 -- F3_CB_4/LConn3
  SSN Interface Block (3ph)5/RConn5 -- F3_CB_4/LConn2
  C2/LConn1 -- F3_CB_3/LConn1 -- SSN Interface Block (3ph)5/RConn7
  C2/LConn3 -- F3_CB_3/LConn3 -- SSN Interface Block (3ph)5/RConn9
  C2/LConn2 -- F3_CB_3/LConn2 -- SSN Interface Block (3ph)5/RConn8
  C303/LConn1 -- F3_CB_4/RConn1
  C303/LConn2 -- F3_CB_4/RConn2
  C303/LConn3 -- F3_CB_4/RConn3
  C303/RConn2 -- 2500 kVA/LConn2
  C303/RConn3 -- 2500 kVA/LConn3
  C303/RConn1 -- 2500 kVA/LConn1
  1000 kVA1/RConn1 -- Critical_6/LConn1
  1000 kVA1/RConn2 -- Critical_6/LConn2
  1000 kVA1/RConn3 -- Critical_6/LConn3
  500kcmil-Mutual1/RConn2 -- 6 kvar inductor at 480V  to cancel kvar produced by the stublines3/LConn2
  6 kvar inductor at 480V  to cancel kvar produced by the stublines3/LConn1 -- 500kcmil-Mutual1/RConn1
  500kcmil-Mutual1/RConn3 -- 6 kvar inductor at 480V  to cancel kvar produced by the stublines3/LConn3
  500kcmil-Mutual2/RConn2 -- 6 kvar inductor at 480V  to cancel kvar produced by the stublines2/LConn2
  500kcmil-Mutual2/RConn3 -- 6 kvar inductor at 480V  to cancel kvar produced by the stublines2/LConn3
  500kcmil-Mutual2/RConn1 -- 6 kvar inductor at 480V  to cancel kvar produced by the stublines2/LConn1
  500kcmil-Mutual4/RConn2 -- 6 kvar inductor at 480V  to cancel kvar produced by the stublines1/LConn2
  500kcmil-Mutual4/RConn3 -- 6 kvar inductor at 480V  to cancel kvar produced by the stublines1/LConn3
  500kcmil-Mutual4/RConn1 -- 6 kvar inductor at 480V  to cancel kvar produced by the stublines1/LConn1
  500kcmil-Mutual3/LConn3 -- F3_PCC/RConn3
  500kcmil-Mutual3/LConn1 -- F3_PCC/RConn1
  500kcmil-Mutual3/LConn2 -- F3_PCC/RConn2
  500kcmil-Mutual5/RConn1 -- F3_PCC/LConn1
  500kcmil-Mutual5/RConn2 -- F3_PCC/LConn2
  500kcmil-Mutual5/RConn3 -- F3_PCC/LConn3
  500kcmil-Mutual4/LConn3 -- 1000 kVA/RConn3 -- F3_CB_11/LConn3
  C1/RConn2 -- SSN Interface Block (3ph)1/LConn2
  C1/RConn3 -- SSN Interface Block (3ph)1/LConn3
  C1/RConn1 -- SSN Interface Block (3ph)1/LConn1
  500kcmil-Mutual3/RConn1 -- SSN Interface Block (3ph)5/LConn1 -- Losses4/LConn1
  500kcmil-Mutual3/RConn2 -- SSN Interface Block (3ph)5/LConn2 -- Losses4/LConn2
  500kcmil-Mutual3/RConn3 -- SSN Interface Block (3ph)5/LConn3 -- Losses4/LConn3
  PCC_A/RConn1 -- 500kcmil-Mutual5/LConn1 -- 448 kvar inductor at 13.8kV  to cancel kvar produced by the stublines1/LConn1
  PCC_B/RConn1 -- 448 kvar inductor at 13.8kV  to cancel kvar produced by the stublines1/LConn2 -- 500kcmil-Mutual5/LConn2
  PCC_C/RConn1 -- 448 kvar inductor at 13.8kV  to cancel kvar produced by the stublines1/LConn3 -- 500kcmil-Mutual5/LConn3
  SSN Interface Block (3ph)2/RConn3 -- F3_CB_2/LConn3
  SSN Interface Block (3ph)2/RConn2 -- F3_CB_2/LConn2
  SSN Interface Block (3ph)2/RConn1 -- F3_CB_2/LConn1
  C2/RConn2 -- SSN Interface Block (3ph)2/LConn2
  C2/RConn1 -- SSN Interface Block (3ph)2/LConn1
  C2/RConn3 -- SSN Interface Block (3ph)2/LConn3
  F3_CB_1/LConn2 -- SSN Interface Block (3ph)5/RConn11
  F3_CB_1/LConn1 -- SSN Interface Block (3ph)5/RConn10
  F3_CB_1/LConn3 -- SSN Interface Block (3ph)5/RConn12
  SSN Interface Block (3ph)1/RConn1 -- F3_CB_6/LConn1
  SSN Interface Block (3ph)1/RConn2 -- F3_CB_6/LConn2
  SSN Interface Block (3ph)1/RConn3 -- F3_CB_6/LConn3
  F3_CB_1/RConn1 -- C301/LConn1
  F3_CB_1/RConn2 -- C301/LConn2
  F3_CB_1/RConn3 -- C301/LConn3
  F3_CB_10/LConn3 -- SSN Interface Block (3ph)5/RConn3
  F3_CB_10/LConn2 -- SSN Interface Block (3ph)5/RConn2
  F3_CB_10/LConn1 -- SSN Interface Block (3ph)5/RConn1
  2500 kVA1/LConn2 -- F3_CB_10/RConn2
  2500 kVA1/LConn1 -- F3_CB_10/RConn1
  2500 kVA1/LConn3 -- F3_CB_10/RConn3
  PHIL_F3/LConn3 -- 2500 kVA1/RConn3
  PHIL_F3/LConn2 -- 2500 kVA1/RConn2
  PHIL_F3/LConn1 -- 2500 kVA1/RConn1

== system Ghost_f34/SC_ctrl/CB_modbus_mock ==
  note: Should be from pattern generator
  Bus Creator1 : BusCreator  Inputs=7
  Enabled : Constant
  F1 : Subsystem
  F2 : Subsystem
  F3 : Subsystem
  F4 : Subsystem
  Manual Switch{,1..3} (4 alike) : ManualSwitch
  Manual Switch4 : ManualSwitch  CurrentSetting=0
  NO FAULT : Constant  Value=0
  NO FAULT2 : Constant  Value=0
  NO FAULT3 : Constant  Value=0
  Pulse Generator : DiscretePulseGenerator  SampleTime=[Stim.Ts Ts]
  RST : Constant
  Rate Transition : RateTransition  Deterministic=off
  setting #1 : Constant  Value=0
  setting #2 : Constant
  Out1 : Outport
  wires:
  Bus Creator1/1 -> Rate Transition/1
  F4/1(Out1) -> Bus Creator1/4  "F4"
  F3/1(Out1) -> Bus Creator1/3  "F3"
  F2/1(Out1) -> Bus Creator1/2  "F2"
  F1/1(Out1) -> Bus Creator1/1  "F1"
  Manual Switch/1 -> Bus Creator1/5  "ResetAll"
  Manual Switch1/1 -> Manual Switch/2
  Pulse Generator/1 -> Manual Switch/1
  NO FAULT/1 -> Manual Switch1/1
  RST/1 -> Manual Switch1/2  "record_rms_signals"
  Manual Switch3/1 -> Manual Switch2/2
  NO FAULT2/1 -> Manual Switch2/1
  setting #1/1 -> Manual Switch3/1
  setting #2/1 -> Manual Switch3/2  "record_rms_signals"
  Manual Switch2/1 -> Bus Creator1/6  "GroupSel"
  Manual Switch4/1 -> Bus Creator1/7  "MockEna"
  NO FAULT3/1 -> Manual Switch4/1
  Enabled/1 -> Manual Switch4/2  "record_rms_signals"
  Rate Transition/1 -> Out1/1

== system Ghost_f34/SC_ctrl/Gen1_Modbus_Stimuli2 ==
  note: Use Modbus from
      | Console
  note: Use Modbus TCP
  Bus Creator1 : BusCreator  Inputs=2
  Bus Creator12 : BusCreator  Inputs=8
  Fcmd pu : Constant  Value=1.003
  Gain3 : Gain  Gain=4000
  Gain4 : Gain  Gain=4000
  Gain5 : Gain  Gain=13800
  Gain6 : Gain  Gain=6000
  Manual Switch2 : ManualSwitch
  Manual Switch3 : ManualSwitch
  Manual Switch4 : ManualSwitch
  PCmd1 : Constant  Value=300
  PCmd2 : Constant  Value=300
  PCmd3 : Constant  Value=0
  PCmd4 : Constant  Value=0
  PCmd5 : Constant  Value=12
  PCmd6 : Constant  Value=0
  PCmd7 : Constant
  PCmd8 : Constant  Value=11
  Pfactor : Gain  Gain=.9
  Qfactor : Gain  Gain=.43
  Rate Transition1 : RateTransition  Deterministic=off
  S Profile3 : simulink/Sources/Repeating Sequence Stair  OutValues=Stim.Gen3.s  tsamp=[Stim.Ts Ts]  OutMin=[]  OutMax=[]  OutDataTypeStr=Inherit: Inherit via back propagation  OutDataType=fixdt(0,8)  ConRadixGroup=Best Precision: Vector-wise  OutScaling=2^-12
  Vcmd pu : Constant
  MbCtrl : Outport
  wires:
  S Profile3/1 -> Pfactor/1, Qfactor/1  "P"
  Qfactor/1 -> Manual Switch3/1  "Q"
  Vcmd pu/1 -> Gain5/1  "V"
  Fcmd pu/1 -> Gain6/1  "F"
  Pfactor/1 -> Manual Switch2/1  "P"
  Manual Switch2/1 -> Gain3/1
  Bus Creator12/1 -> Bus Creator1/1  "ModbusFromSC"
  Manual Switch3/1 -> Gain4/1
  PCmd4/1 -> Manual Switch3/2
  PCmd3/1 -> Manual Switch2/2
  PCmd1/1 -> Bus Creator12/6
  PCmd2/1 -> Bus Creator12/7
  PCmd5/1 -> Bus Creator12/8
  Bus Creator1/1 -> Rate Transition1/1
  Manual Switch4/1 -> Bus Creator1/2  "ModbusEnable"
  PCmd6/1 -> Manual Switch4/1
  PCmd7/1 -> Manual Switch4/2
  Gain3/1 -> Bus Creator12/2  "PCmd"
  Gain4/1 -> Bus Creator12/3  "QCmd"
  Gain5/1 -> Bus Creator12/4  "VoltCmd"
  Gain6/1 -> Bus Creator12/5  "FreqCmd"
  Rate Transition1/1 -> MbCtrl/1
  PCmd8/1 -> Bus Creator12/1  "Ctrl"

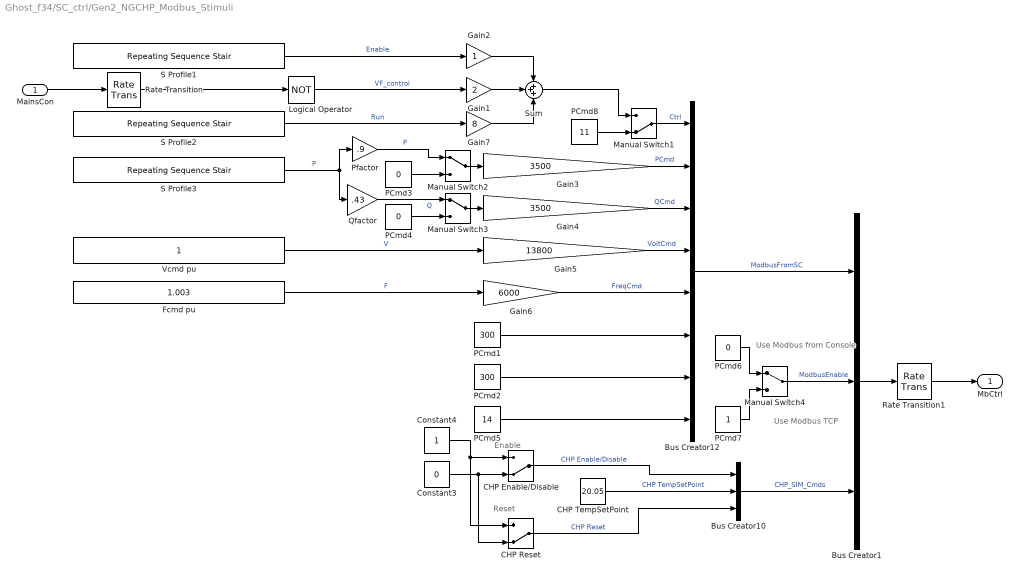
== system Ghost_f34/SC_ctrl/Gen2_NGCHP_Modbus_Stimuli ==
  note: Use Modbus TCP
  note: Use Modbus from
      | Console
  note: Enable
  note: Reset
  MainsCon : Inport
  Bus Creator1 : BusCreator  Inputs=3
  Bus Creator10 : BusCreator  Inputs=3
  Bus Creator12 : BusCreator  Inputs=8
  CHP Enable/Disable : ManualSwitch  CurrentSetting=0
  CHP Reset : ManualSwitch  CurrentSetting=0
  CHP TempSetPoint : Constant  Value=20.05
  Constant3 : Constant  Value=0
  Constant4 : Constant
  Fcmd pu : Constant  Value=1.003
  Gain1 : Gain  Gain=2  OutDataTypeStr=double
  Gain2 : Gain
  Gain3 : Gain  Gain=3500
  Gain4 : Gain  Gain=3500
  Gain5 : Gain  Gain=13800
  Gain6 : Gain  Gain=6000
  Gain7 : Gain  Gain=8
  Logical Operator : Logic  Operator=NOT  AllPortsSameDT=off  OutDataTypeStr=boolean
  Manual Switch1 : ManualSwitch  CurrentSetting=0
  Manual Switch2 : ManualSwitch
  Manual Switch3 : ManualSwitch
  Manual Switch4 : ManualSwitch
  PCmd1 : Constant  Value=300
  PCmd2 : Constant  Value=300
  PCmd3 : Constant  Value=0
  PCmd4 : Constant  Value=0
  PCmd5 : Constant  Value=14
  PCmd6 : Constant  Value=0
  PCmd7 : Constant
  PCmd8 : Constant  Value=11
  Pfactor : Gain  Gain=.9
  Qfactor : Gain  Gain=.43
  Rate Transition : RateTransition  Deterministic=off
  Rate Transition1 : RateTransition  Deterministic=off
  S Profile1 : simulink/Sources/Repeating Sequence Stair  OutValues=Stim.Gen3.Ena  tsamp=[Stim.Ts Ts]  OutMin=[]  OutMax=[]  OutDataTypeStr=Inherit: Inherit via back propagation  OutDataType=fixdt(0,8)  ConRadixGroup=Best Precision: Vector-wise  OutScaling=2^-12
  S Profile2 : simulink/Sources/Repeating Sequence Stair  OutValues=Stim.Gen3.Run  tsamp=[Stim.Ts Ts]  OutMin=[]  OutMax=[]  OutDataTypeStr=Inherit: Inherit via back propagation  OutDataType=fixdt(0,8)  ConRadixGroup=Best Precision: Vector-wise  OutScaling=2^-12
  S Profile3 : simulink/Sources/Repeating Sequence Stair  OutValues=Stim.Gen3.s  tsamp=[Stim.Ts Ts]  OutMin=[]  OutMax=[]  OutDataTypeStr=Inherit: Inherit via back propagation  OutDataType=fixdt(0,8)  ConRadixGroup=Best Precision: Vector-wise  OutScaling=2^-12
  Sum : Sum  Inputs=+++
  Vcmd pu : Constant
  MbCtrl : Outport
  wires:
  Rate Transition/1 -> Logical Operator/1
  Logical Operator/1 -> Gain1/1  "VF_control"
  MainsCon/1 -> Rate Transition/1
  Gain7/1 -> Sum/3
  S Profile2/1 -> Gain7/1  "Run"
  Gain6/1 -> Bus Creator12/5  "FreqCmd"
  Gain5/1 -> Bus Creator12/4  "VoltCmd"
  Gain4/1 -> Bus Creator12/3  "QCmd"
  Gain3/1 -> Bus Creator12/2  "PCmd"
  PCmd7/1 -> Manual Switch4/2
  PCmd6/1 -> Manual Switch4/1
  Manual Switch4/1 -> Bus Creator1/2  "ModbusEnable"
  Bus Creator1/1 -> Rate Transition1/1
  PCmd5/1 -> Bus Creator12/8
  PCmd2/1 -> Bus Creator12/7
  PCmd1/1 -> Bus Creator12/6
  Sum/1 -> Manual Switch1/1
  Gain1/1 -> Sum/2
  Gain2/1 -> Sum/1
  PCmd3/1 -> Manual Switch2/2
  PCmd4/1 -> Manual Switch3/2
  Manual Switch3/1 -> Gain4/1
  Bus Creator12/1 -> Bus Creator1/1  "ModbusFromSC"
  Manual Switch2/1 -> Gain3/1
  S Profile1/1 -> Gain2/1  "Enable"
  Pfactor/1 -> Manual Switch2/1  "P"
  Fcmd pu/1 -> Gain6/1  "F"
  Vcmd pu/1 -> Gain5/1  "V"
  Qfactor/1 -> Manual Switch3/1  "Q"
  S Profile3/1 -> Qfactor/1, Pfactor/1  "P"
  Bus Creator10/1 -> Bus Creator1/3  "CHP_SIM_Cmds"
  CHP Reset/1 -> Bus Creator10/3  "CHP Reset"
  CHP TempSetPoint/1 -> Bus Creator10/2  "CHP TempSetPoint"
  CHP Enable/Disable/1 -> Bus Creator10/1  "CHP Enable/Disable"
  Constant4/1 -> CHP Enable/Disable/1, CHP Reset/1
  Constant3/1 -> CHP Enable/Disable/2, CHP Reset/2
  Rate Transition1/1 -> MbCtrl/1
  PCmd8/1 -> Manual Switch1/2
  Manual Switch1/1 -> Bus Creator12/1  "Ctrl"

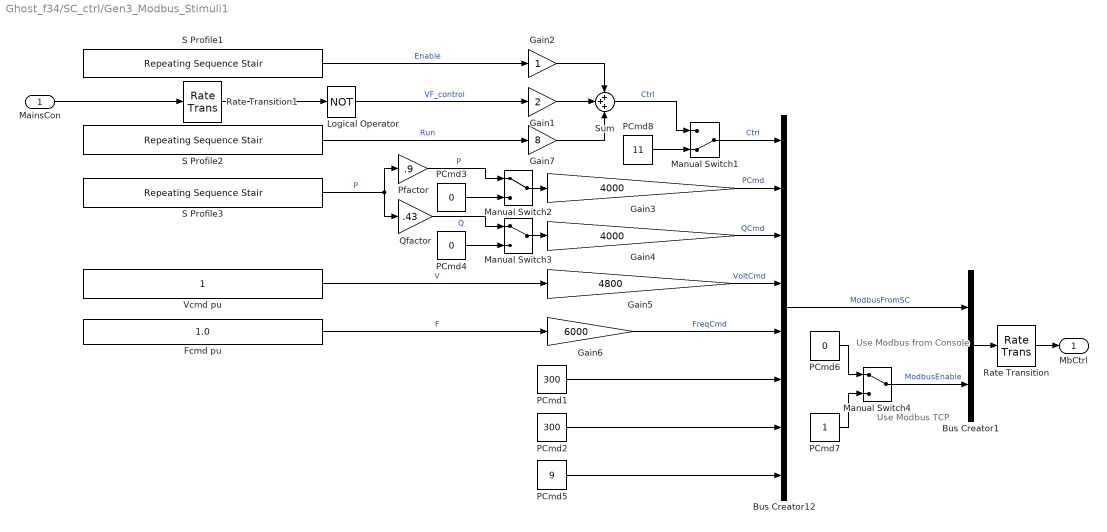
== system Ghost_f34/SC_ctrl/Gen3_Modbus_Stimuli1 ==
  note: Use Modbus TCP
  note: Use Modbus from
      | Console
  MainsCon : Inport
  Bus Creator1 : BusCreator  Inputs=2
  Bus Creator12 : BusCreator  Inputs=8
  Fcmd pu : Constant  Value=1.0
  Gain1 : Gain  Gain=2  OutDataTypeStr=double
  Gain2 : Gain
  Gain3 : Gain  Gain=4000
  Gain4 : Gain  Gain=4000
  Gain5 : Gain  Gain=4800
  Gain6 : Gain  Gain=6000
  Gain7 : Gain  Gain=8
  Logical Operator : Logic  Operator=NOT  AllPortsSameDT=off  OutDataTypeStr=boolean
  Manual Switch1 : ManualSwitch  CurrentSetting=0
  Manual Switch2 : ManualSwitch
  Manual Switch3 : ManualSwitch
  Manual Switch4 : ManualSwitch
  PCmd1 : Constant  Value=300
  PCmd2 : Constant  Value=300
  PCmd3 : Constant  Value=0
  PCmd4 : Constant  Value=0
  PCmd5 : Constant  Value=9
  PCmd6 : Constant  Value=0
  PCmd7 : Constant
  PCmd8 : Constant  Value=11
  Pfactor : Gain  Gain=.9
  Qfactor : Gain  Gain=.43
  Rate Transition : RateTransition  Deterministic=off
  Rate Transition1 : RateTransition  Deterministic=off
  S Profile1 : simulink/Sources/Repeating Sequence Stair  OutValues=Stim.Gen3.Ena  tsamp=[Stim.Ts Ts]  OutMin=[]  OutMax=[]  OutDataTypeStr=Inherit: Inherit via back propagation  OutDataType=fixdt(0,8)  ConRadixGroup=Best Precision: Vector-wise  OutScaling=2^-12
  S Profile2 : simulink/Sources/Repeating Sequence Stair  OutValues=Stim.Gen3.Run  tsamp=[Stim.Ts Ts]  OutMin=[]  OutMax=[]  OutDataTypeStr=Inherit: Inherit via back propagation  OutDataType=fixdt(0,8)  ConRadixGroup=Best Precision: Vector-wise  OutScaling=2^-12
  S Profile3 : simulink/Sources/Repeating Sequence Stair  OutValues=Stim.Gen3.s  tsamp=[Stim.Ts Ts]  OutMin=[]  OutMax=[]  OutDataTypeStr=Inherit: Inherit via back propagation  OutDataType=fixdt(0,8)  ConRadixGroup=Best Precision: Vector-wise  OutScaling=2^-12
  Sum : Sum  Inputs=+++
  Vcmd pu : Constant
  MbCtrl : Outport
  wires:
  MainsCon/1 -> Rate Transition1/1
  Logical Operator/1 -> Gain1/1  "VF_control"
  Gain7/1 -> Sum/3
  S Profile2/1 -> Gain7/1  "Run"
  Gain6/1 -> Bus Creator12/5  "FreqCmd"
  Gain5/1 -> Bus Creator12/4  "VoltCmd"
  Gain4/1 -> Bus Creator12/3  "QCmd"
  Gain3/1 -> Bus Creator12/2  "PCmd"
  PCmd7/1 -> Manual Switch4/2
  PCmd6/1 -> Manual Switch4/1
  Manual Switch4/1 -> Bus Creator1/2  "ModbusEnable"
  Bus Creator1/1 -> Rate Transition/1
  PCmd5/1 -> Bus Creator12/8
  PCmd2/1 -> Bus Creator12/7
  PCmd1/1 -> Bus Creator12/6
  Sum/1 -> Manual Switch1/1  "Ctrl"
  Gain1/1 -> Sum/2
  Gain2/1 -> Sum/1
  PCmd3/1 -> Manual Switch2/2
  PCmd4/1 -> Manual Switch3/2
  Manual Switch3/1 -> Gain4/1
  Bus Creator12/1 -> Bus Creator1/1  "ModbusFromSC"
  Manual Switch2/1 -> Gain3/1
  S Profile1/1 -> Gain2/1  "Enable"
  Pfactor/1 -> Manual Switch2/1  "P"
  Fcmd pu/1 -> Gain6/1  "F"
  Vcmd pu/1 -> Gain5/1  "V"
  Qfactor/1 -> Manual Switch3/1  "Q"
  S Profile3/1 -> Qfactor/1, Pfactor/1  "P"
  Rate Transition/1 -> MbCtrl/1
  Rate Transition1/1 -> Logical Operator/1
  PCmd8/1 -> Manual Switch1/2
  Manual Switch1/1 -> Bus Creator12/1  "Ctrl"
